simulink model "Nonlinear_Fixedpoint"  (R2018a)
settings: Solver=VariableStepAuto  StartTime=0.0  StopTime=30  MaxStep=0.01  RelTol=1e-3
values from neighbouring files (symbols this model uses):
  g = 9.80665    [CPscript_friction.m]    (also in fixedptscript_R0.m)
  KD = [(F_i/omega_i) (F_i*alpha_0/alpha_i) F_i/vel_i  F_i/x_i].*(kt_dg)    [CPscript_friction.m]    (also in fixedptscript_R0.m)
  kd_i = [omega_i 0 0 0 ; 0 (alpha_i/alpha_0) 0 0 ; 0 0 vel_i 0 ; 0 0 0 (x_i/x_0)]    [CPscript_friction.m]    (also in fixedptscript_R0.m)
  KI_D = (x_0/x_i)* ki_d *(F_i/F_0)    [CPscript_friction.m]    (also in fixedptscript_R0.m)
  KP_D = (x_0/x_i)* p *(F_i/F_0)    [CPscript_friction.m]    (also in fixedptscript_R0.m)
  l = 0.285    [CPscript_friction.m]    (also in fixedptscript_R0.m)
  M = 4.676    [CPscript_friction.m]    (also in fixedptscript_R0.m)
  m = 0.098    [CPscript_friction.m]    (also in fixedptscript_R0.m)
  Phyval = F_0/F_i    (= 0.0453448932581)    [CPscript_friction.m]    (also in fixedptscript_R0.m)
  Ts = 10e-3    (= 0.01)    [CPscript_friction.m]    (also in fixedptscript_R0.m)
  x_i = 28619    [CPscript_friction.m]    (also in fixedptscript_R0.m)
settings Model: Creator=govardan  LastModifiedBy=govardan

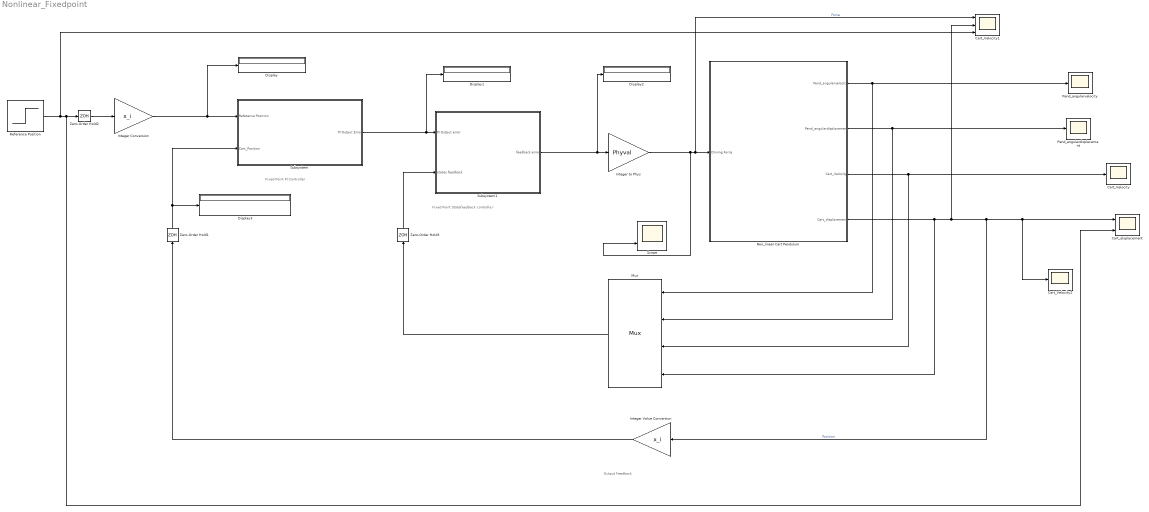
== system Nonlinear_Fixedpoint ==
  note: Output Feedback
  note: Fixed Point Statefeedback controlle r
  note: Fixed Point PI Controller
  Cart_Velocity : Scope
  Cart_Velocity1 : Scope  NumInputPorts=3
  Cart_Velocity2 : Scope
  Cart_displacement : Scope  NumInputPorts=2
  Display{,1..3} (4 alike) : Display
  Integer Conversion : Gain  Gain=x_i  ParamDataTypeStr=fixdt(1,16,0)  OutDataTypeStr=fixdt(1,16,0)
  Integer Value Conversion : Gain  Gain=x_i  ParamDataTypeStr=int16  OutDataTypeStr=int16
  Integer to Phys : Gain  Gain=Phyval  ParamDataTypeStr=fixdt(1,32,9)  OutDataTypeStr=fixdt(1,32,9)
  Mux : Mux
      settings: DisplayOption=signals
  Non_linear Cart Pendulum : Subsystem
  Pend_angulardisplacement : Scope
  Pend_angularvelocity : Scope
  Reference Position : Step  SampleTime=0
  Scope : Scope  NumInputPorts=2
  Subsystem : Subsystem
  Subsystem1 : Subsystem
  Zero-Order Hold1 : ZeroOrderHold  SampleTime=-1
  Zero-Order Hold2 : ZeroOrderHold  SampleTime=-1
  Zero-Order Hold3 : ZeroOrderHold  SampleTime=-1
  wires:
  Non_linear Cart Pendulum/1("                   Pend_angularvelocity") -> Mux/1, Pend_angularvelocity/1
  Integer Value Conversion/1 -> Zero-Order Hold1/1
  Reference Position/1 -> Cart_Velocity1/3, Cart_displacement/2, Zero-Order Hold2/1
  Non_linear Cart Pendulum/2("                   Pend_angulardisplacement") -> Mux/2, Pend_angulardisplacement/1
  Non_linear Cart Pendulum/3(Cart_Velocity) -> Mux/3, Cart_Velocity/1
  Zero-Order Hold2/1 -> Integer Conversion/1
  Integer Conversion/1 -> Display/1, Subsystem/1(Refetence Position)
  Subsystem1/1(feedback error) -> Display2/1, Integer to Phys/1
  Subsystem/1(PI Output Error) -> Display1/1, Subsystem1/1(PI Output error)
  Non_linear Cart Pendulum/4(Cart_displacement) -> Mux/4, Cart_Velocity1/2, Integer Value Conversion/1, Cart_Velocity2/1, Cart_displacement/1  "Position"
  Integer to Phys/1 -> Scope/2, Cart_Velocity1/1, Non_linear Cart Pendulum/1(Driving Force)  "Force"
  Zero-Order Hold1/1 -> Subsystem/2(Cart_Position), Display3/1
  Mux/1 -> Zero-Order Hold3/1
  Zero-Order Hold3/1 -> Subsystem1/2(states feedback)

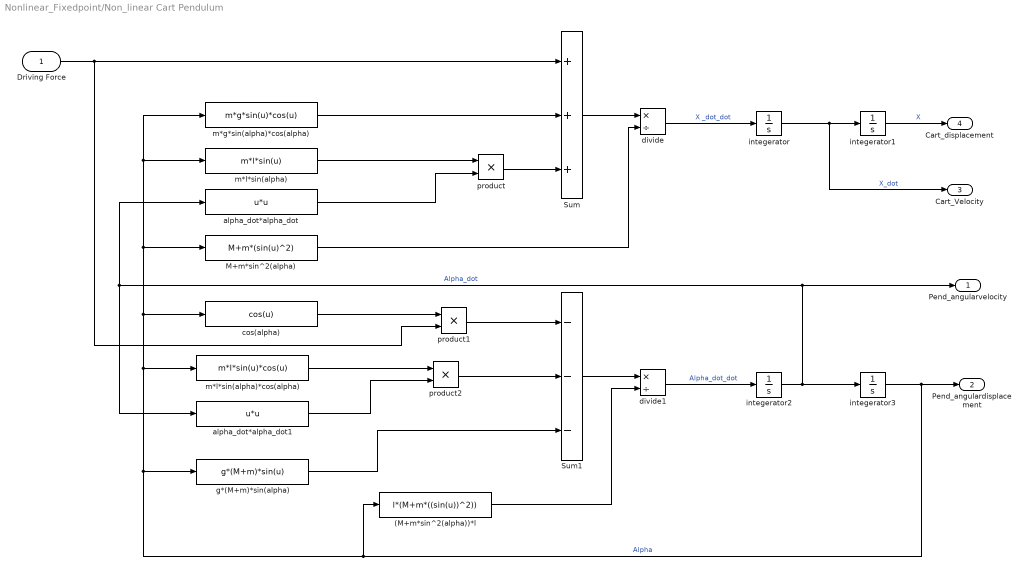
== system Nonlinear_Fixedpoint/Non_linear Cart Pendulum ==
  Driving Force : Inport
  (M+m*sin^2(alpha))*l : Fcn  Expr=l*(M+m*((sin(u))^2))
  M+m*sin^2(alpha) : Fcn  Expr=M+m*(sin(u)^2)
  Sum : Sum  Inputs=+++
  Sum1 : Sum  Inputs=---
  alpha_dot*alpha_dot : Fcn  Expr=u*u
  alpha_dot*alpha_dot1 : Fcn  Expr=u*u
  cos(alpha) : Fcn  Expr=cos(u)
  divide : Product  Inputs=*/
  divide1 : Product  Inputs=*/
  g*(M+m)*sin(alpha) : Fcn  Expr=g*(M+m)*sin(u)
  integerator{,1..3} (4 alike) : Integrator
  m*g*sin(alpha)*cos(alpha) : Fcn  Expr=m*g*sin(u)*cos(u)
  m*l*sin(alpha) : Fcn  Expr=m*l*sin(u)
  m*l*sin(alpha)*cos(alpha) : Fcn  Expr=m*l*sin(u)*cos(u)
  product : Product
  product1 : Product
  product2 : Product
  "                   Pend_angularvelocity" : Outport
  "                   Pend_angulardisplacement" : Outport  Port=2
  Cart_Velocity : Outport  Port=3
  Cart_displacement : Outport  Port=4
  wires:
  product1/1 -> Sum1/1
  Driving Force/1 -> Sum/1, product1/2
  divide1/1 -> integerator2/1  "Alpha_dot_dot"
  cos(alpha)/1 -> product1/1
  m*g*sin(alpha)*cos(alpha)/1 -> Sum/2
  integerator1/1 -> Cart_displacement/1  "X"
  integerator2/1 -> integerator3/1, "                   Pend_angularvelocity"/1, alpha_dot*alpha_dot1/1, alpha_dot*alpha_dot/1  "Alpha_dot"
  integerator/1 -> Cart_Velocity/1, integerator1/1  "X_dot"
  Sum/1 -> divide/1
  integerator3/1 -> "                   Pend_angulardisplacement"/1, g*(M+m)*sin(alpha)/1, m*l*sin(alpha)*cos(alpha)/1, cos(alpha)/1, M+m*sin^2(alpha)/1, m*l*sin(alpha)/1, m*g*sin(alpha)*cos(alpha)/1, (M+m*sin^2(alpha))*l/1  "Alpha"
  divide/1 -> integerator/1  "X _dot_dot"
  m*l*sin(alpha)*cos(alpha)/1 -> product2/1
  g*(M+m)*sin(alpha)/1 -> Sum1/3
  m*l*sin(alpha)/1 -> product/1
  alpha_dot*alpha_dot/1 -> product/2
  M+m*sin^2(alpha)/1 -> divide/2
  alpha_dot*alpha_dot1/1 -> product2/2
  product/1 -> Sum/3
  (M+m*sin^2(alpha))*l/1 -> divide1/2
  Sum1/1 -> divide1/1
  product2/1 -> Sum1/2

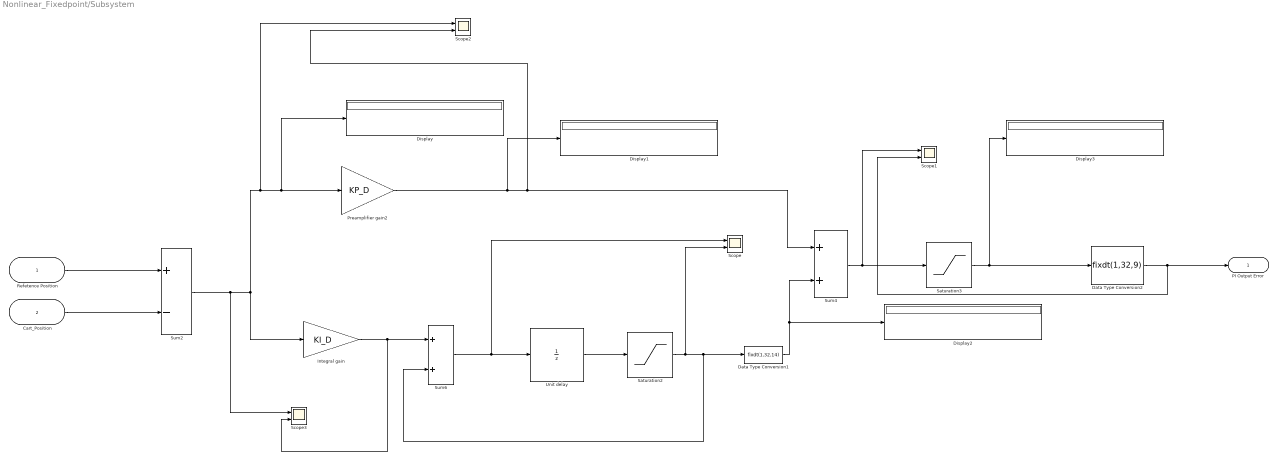
== system Nonlinear_Fixedpoint/Subsystem ==
  Refetence Position : Inport
  Cart_Position : Inport  Port=2
  Data Type Conversion1 : DataTypeConversion  OutDataTypeStr=fixdt(1,32,14)
  Data Type Conversion2 : DataTypeConversion  OutDataTypeStr=fixdt(1,32,9)
  Display{,1..3} (4 alike) : Display
      settings: Format=long_e
  Integral gain : Gain  Gain=KI_D  ParamDataTypeStr=fixdt(1,16,15)
  Preamplifier gain2 : Gain  Gain=KP_D  ParamDataTypeStr=fixdt(1,16,14)
  Saturation2 : Saturate  UpperLimit=32768  LowerLimit=-32768
  Saturation3 : Saturate  UpperLimit=16384  LowerLimit=-16384
  Scope{,1..3} (4 alike) : Scope  NumInputPorts=2
  Sum2 : Sum  Inputs=+-
  Sum4 : Sum
  Sum6 : Sum  AccumDataTypeStr=fixdt(1,50,14)
  Unit delay : UnitDelay  SampleTime=Ts
  PI Output Error : Outport
  wires:
  Sum2/1 -> Scope3/1, Integral gain/1, Scope2/1, Display/1, Preamplifier gain2/1
  Integral gain/1 -> Scope3/2, Sum6/1
  Unit delay/1 -> Saturation2/1
  Data Type Conversion2/1 -> Scope1/2, PI Output Error/1
  Refetence Position/1 -> Sum2/1
  Cart_Position/1 -> Sum2/2
  Data Type Conversion1/1 -> Sum4/2, Display2/1
  Sum6/1 -> Scope/1, Unit delay/1
  Saturation2/1 -> Scope/2, Data Type Conversion1/1, Sum6/2
  Preamplifier gain2/1 -> Display1/1, Scope2/2, Sum4/1
  Sum4/1 -> Scope1/1, Saturation3/1
  Saturation3/1 -> Display3/1, Data Type Conversion2/1

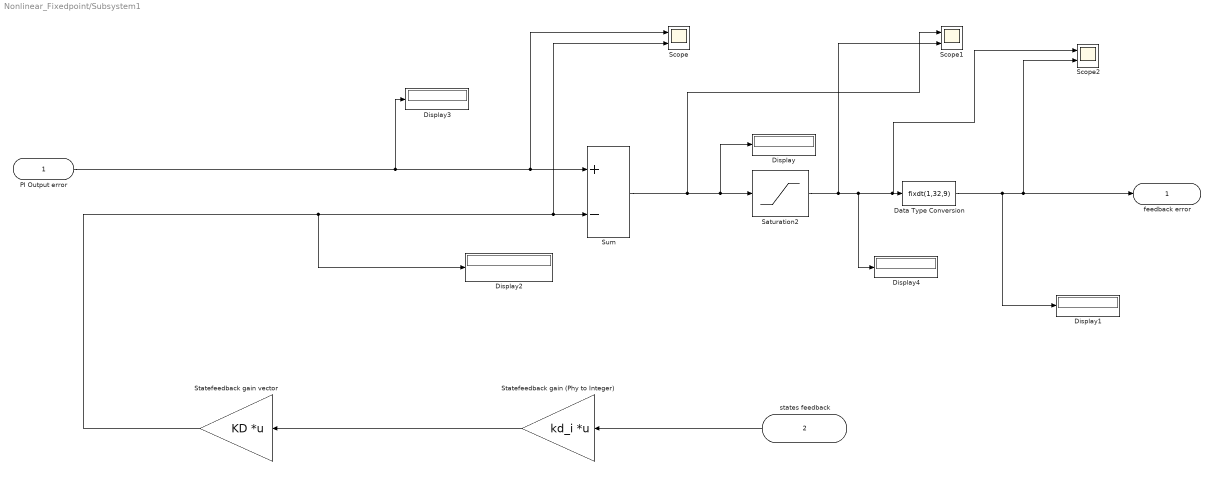
== system Nonlinear_Fixedpoint/Subsystem1 ==
  PI Output error : Inport
  states feedback : Inport  Port=2
  Data Type Conversion : DataTypeConversion  OutDataTypeStr=fixdt(1,32,9)
  Display{,1..4} (5 alike) : Display
  Saturation2 : Saturate  UpperLimit=1048064  LowerLimit=-1048064
  Scope : Scope  NumInputPorts=2
  Scope1 : Scope  NumInputPorts=2
  Scope2 : Scope  NumInputPorts=2
  Statefeedback gain (Phy to Integer) : Gain  Gain=kd_i  Multiplication=Matrix(K*u) (u vector)  ParamDataTypeStr=int16  OutDataTypeStr=int16
  Statefeedback gain vector : Gain  Gain=KD  Multiplication=Matrix(K*u) (u vector)  ParamDataTypeStr=fixdt(1,16,9)
  Sum : Sum  Inputs=+-
  feedback error : Outport
  wires:
  Sum/1 -> Scope1/1, Display/1, Saturation2/1
  Statefeedback gain (Phy to Integer)/1 -> Statefeedback gain vector/1
  PI Output error/1 -> Scope/1, Sum/1, Display3/1
  states feedback/1 -> Statefeedback gain (Phy to Integer)/1
  Data Type Conversion/1 -> Scope2/2, feedback error/1, Display1/1
  Saturation2/1 -> Scope1/2, Display4/1, Scope2/1, Data Type Conversion/1
  Statefeedback gain vector/1 -> Display2/1, Scope/2, Sum/2
